simulink model "simulazione"  (R2023a)
settings: Solver=FixedStepAuto  StartTime=0.0  StopTime=10  FixedStep=1e-3  RelTol=1e-3
settings Model: Creator=effi  LastModifiedBy=effi

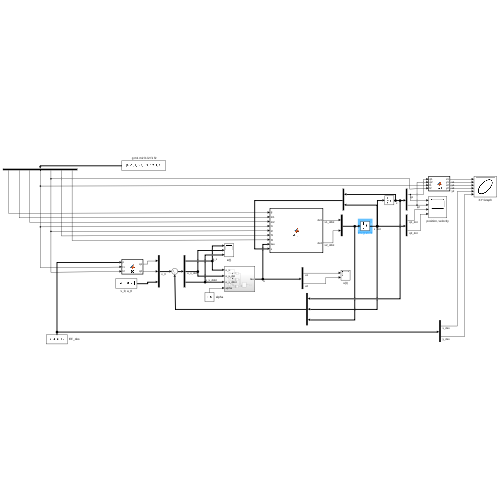
[thumbnail: Simulink's stored preview of the top-level diagram]
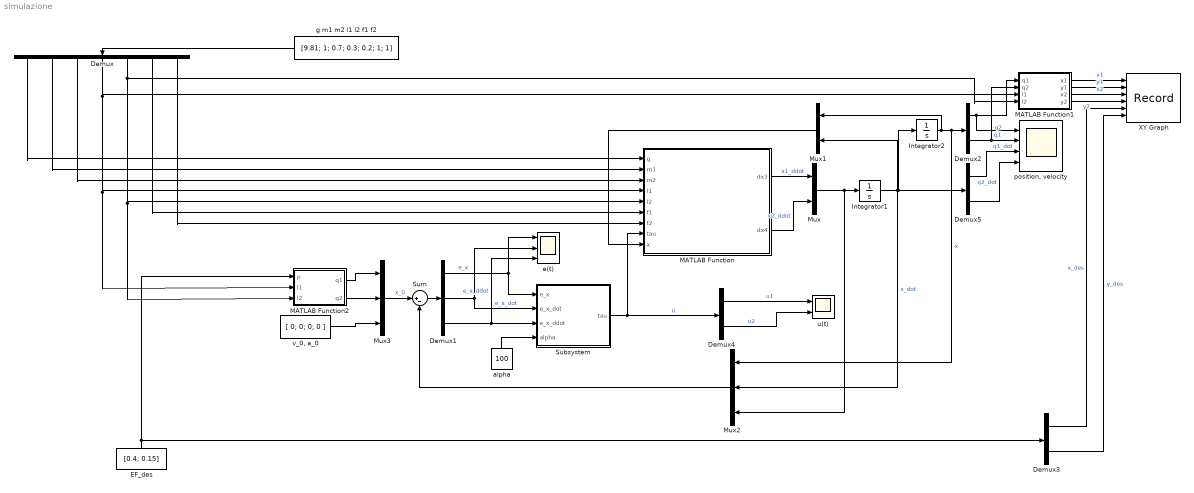
== system simulazione ==
  " g m1 m2 l1 l2 f1 f2" : Constant  Value=[9.81; 1; 0.7; 0.3; 0.2; 1; 1]  SampleTime=-1
  Demux : Demux  Outputs=7
  Demux1 : Demux  Outputs=3
  Demux{2..5} (4 alike) : Demux  Outputs=2
  EF_des : Constant  Value=[0.4; 0.15]  SampleTime=-1
  Integrator1 : Integrator  LimitOutput=on  UpperSaturationLimit=[1;1]*pi/180*20  LowerSaturationLimit=[-1,-1]*pi/180*20
  Integrator2 : Integrator  LimitOutput=on  UpperSaturationLimit=[pi; 5/6*pi]  LowerSaturationLimit=[-pi; -5/6*pi]
  MATLAB Function : MATLAB Function  TreatAsAtomicUnit=on
  MATLAB Function1 : MATLAB Function  TreatAsAtomicUnit=on
  MATLAB Function2 : MATLAB Function  TreatAsAtomicUnit=on
  Mux : Mux  Inputs=2
  Mux1 : Mux  Inputs=2
  Mux2 : Mux  Inputs=3
  Mux3 : Mux  Inputs=3
  Subsystem : Subsystem
  Sum : Sum  Inputs=|+-
  XY Graph : Record  FileSettingsInternal="{\"entries\":[{\"content\":{\"excelSettings\":{\"content\":{},\"type\":\"Streamout.ExcelSettings\"}},\"type\":\"Streamout.FileSettingStorage\",\"uuid\":\"\"}],\"packageUris\":[\"http:\\/\\/schema.mathworks.com\\/mf0\\/streamout_blocks\\/R2020a\"],\"version\":\"1.0\"}"  Layout=[1 1]  SignalsInternal="{\"entries\":[{\"content\":{\"signals\":[{\"content\":{\"blockPath\":[],\"dimensions\":[1],\"domain\":\"\",\"lineColor\":\"#a2142f\",\"plots\":[1],\"port\":1,\"sid\":[\"\"],\"signalID\":10315,\"signalName\":\"x1\"},\"type\":\"RecordBlkView.Signal\",\"uuid\":\"\"},{\"content\":{\"blockPath\":[],\"dimensions\":[1],\"domain\":\"\",\"lineColor\":\"#139fff\",\"plots\":[1],\"port\":2,\"sid\":[\"\"],\"signalID\":10319,\"signalName\":\"y1\"},\"type\":\"RecordBlkView.Signal\",\"uuid\":\"\"},{\"content\":{\"blockPath\":[],\"dimensions\":[1],\"domain\":\"\",\"lineColor\":\"#edb120\",\"plots\":[1],\"port\":3,\"sid\":[\"\"],\"signalID\":10323,\"signalName\":\"x2\"},\"type\":\"RecordBlkView.Signal\",\"uuid\":\"\"},{\"content\":{\"blockPath\":[],\"dimensions\":[1],\"domain\":\"\",\"lineColor\":\"#7e2f8e\",\"plots\":[1],\"port\":4,\"sid\":[\"\"],\"signalID\":10327,\"signalName\":\"y2\"},\"type\":\"RecordBlkView.Signal\",\"uuid\":\"\"},{\"content\":{\"blockPath\":[],\"dimensions\":[1],\"domain\":\"\",\"lineColor\":\"#77ac30\",\"plots\":[1],\"port\":5,\"sid\":[\"\"],\"signalID\":10331,\"signalName\":\"x_des\"},\"type\":\"RecordBlkView.Signal\",\"uuid\":\"\"},{\"content\":{\"blockPath\":[],\"dimensions\":[1],\"domain\":\"\",\"lineColor\":\"#4dbeee\",\"plots\":[1],\"port\":6,\"sid\":[\"\"],\"signalID\":10335,\"signalName\":\"y_des\"},\"type\":\"RecordBlkView.Signal\",\"uuid\":\"\"}]},\"type\":\"RecordBlkView.InputSignals\",\"uuid\":\"\"}],\"packageUris\":[\"http:\\/\\/schema.mathworks.com\\/mf0\\/streamout_blocks\\/R2020a\"],\"version\":\"1.0\"}"  VisualizationBindings="{\"xyplotplugin\":{\"info\":[{\"series\":[{\"bindingParametersList\":[{\"parameter\":\"X-Axis\",\"signalID\":10331,\"signalName\":\"x_des\"},{\"parameter\":\"Y-Axis\",\"signalID\":10335,\"signalName\":\"y_des\"}],\"seriesID\":11819},{\"bindingParametersList\":[{\"parameter\":\"X-Axis\",\"signalID\":10323,\"signalName\":\"x2\"},{\"parameter\":\"Y-Axis\",\"signalID\":10327,\"signalName\":\"y2\"}],\"seriesID\":2499},{\"bindingParametersList\":[{\"parameter\":\"X-Axis\",\"signalID\":10315,\"signalName\":\"x1\"},{\"parameter\":\"Y-Axis\",\"signalID\":10319,\"signalName\":\"y1\"}],\"seriesID\":28857}],\"subplotID\":1}]}}"  CompatibilityTag=XY
  alpha : Constant  Value=100
  e(t) : Scope  NumInputPorts=3
  "position, velocity" : Scope  NumInputPorts=4
  u(t) : Scope  NumInputPorts=2
  "v_0, a_0" : Constant  Value=[ 0; 0; 0; 0 ]  SampleTime=-1
  wires:
  Demux3/2 -> XY Graph/6  "y_des"
  MATLAB Function1/4(y2) -> XY Graph/4  "y2"
  MATLAB Function1/2(y1) -> XY Graph/2  "y1"
  Demux3/1 -> XY Graph/5  "x_des"
  MATLAB Function1/1(x1) -> XY Graph/1  "x1"
  Demux5/2 -> "position, velocity"/4  "q2_dot"
  MATLAB Function1/3(x2) -> XY Graph/3  "x2"
  Demux5/1 -> "position, velocity"/3  "q1_dot"
  " g m1 m2 l1 l2 f1 f2"/1 -> Demux/1
  Subsystem/1(tau) -> Demux4/1, MATLAB Function/8(tau)  "u"
  Demux2/2 -> "position, velocity"/2, MATLAB Function1/2(q2)  "q2"
  EF_des/1 -> MATLAB Function2/1(p), Demux3/1
  Demux/7 -> MATLAB Function/7(f2)
  Demux/1 -> MATLAB Function/1(g)
  Demux4/1 -> u(t)/1  "u1"
  MATLAB Function2/2(q2) -> Mux3/2
  "v_0, a_0"/1 -> Mux3/3
  Demux/4 -> MATLAB Function2/2(l1), MATLAB Function/4(l1), MATLAB Function1/3(l1)
  Integrator2/1 -> Demux2/1, Mux2/1, Mux1/1  "x"
  Demux/5 -> MATLAB Function/5(l2), MATLAB Function2/3(l2), MATLAB Function1/4(l2)
  Mux/1 -> Integrator1/1, Mux2/3
  MATLAB Function2/1(q1) -> Mux3/1
  Demux/3 -> MATLAB Function/3(m2)
  Mux3/1 -> Sum/1  "x_0"
  Integrator1/1 -> Integrator2/1, Demux5/1, Mux2/2, Mux1/2  "x_dot"
  Sum/1 -> Demux1/1
  Demux/2 -> MATLAB Function/2(m1)
  Demux1/3 -> e(t)/3, Subsystem/3(e_x_ddot)  "e_x_ddot"
  alpha/1 -> Subsystem/4(alpha)
  Demux1/1 -> e(t)/1, Subsystem/1(e_x)  "e_x"
  Mux2/1 -> Sum/2
  MATLAB Function/1(dx3) -> Mux/1  "x1_ddot"
  Demux4/2 -> u(t)/2  "u2"
  Demux/6 -> MATLAB Function/6(f1)
  MATLAB Function/2(dx4) -> Mux/2  "x2_ddot"
  Mux1/1 -> MATLAB Function/9(x)
  Demux1/2 -> Subsystem/2(e_x_dot), e(t)/2  "e_x_dot"
  Demux2/1 -> MATLAB Function1/1(q1), "position, velocity"/1  "q1"

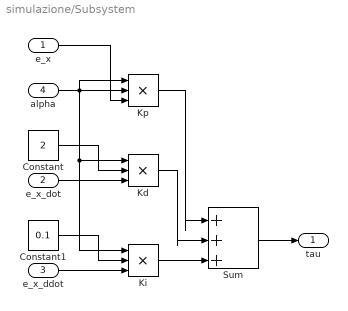
== system simulazione/Subsystem ==
  e_x : Inport
  e_x_dot : Inport  Port=2
  e_x_ddot : Inport  Port=3
  alpha : Inport  Port=4
  Constant : Constant  Value=2
  Constant1 : Constant  Value=0.1
  Kd : Product  Inputs=3
  Ki : Product  Inputs=3
  Kp : Product  Inputs=3
  Sum : Sum  Inputs=|+++
  tau : Outport
  wires:
  Kd/1 -> Sum/2
  Sum/1 -> tau/1
  Constant1/1 -> Ki/2
  Ki/1 -> Sum/3
  e_x_ddot/1 -> Ki/3
  e_x_dot/1 -> Kd/3
  Constant/1 -> Kd/2
  Kp/1 -> Sum/1
  alpha/1 -> Ki/1, Kd/1, Kp/2, Kp/1
  e_x/1 -> Kp/3

== matlab function simulazione/MATLAB Function1 ==
  data: q1 input; x1 output; q2 input; l1 input; l2 input; y1 output; x2 output; y2 output
function [x1,y1,x2,y2] = fwd(q1, q2, l1, l2)

x1 = l1*cos(q1);
y1 = l1*sin(q1);
x2 = x1 + l2*cos(q1+q2);
y2 = y1 + l2*sin(q1+q2);

== matlab function simulazione/MATLAB Function ==
  data: g input; m1 input; m2 input; l1 input; l2 input; f1 input; f2 input; tau input; x input; dx3 output size=1; dx4 output size=1
function [dx3, dx4]  = dxdt(g, m1, m2,l1, l2, f1, f2,tau, x)
    t1 = tau(1);
    t2 = tau(2);
    x1 = x(1);
    x2 = x(2);
    x3 = x(3);
    x4 = x(4);
    % NO FRICTION
    % dx3 = (2*l2*t1 - 2*l2*t2 - 2*l1*t2*cos(x2) - g*l1*l2*m2*cos(x1 + 2*x2) + l1^2*l2*m2*x3^2*sin(2*x2) + 2*l1*l2^2*m2*x3^2*sin(x2) + 2*l1*l2^2*m2*x4^2*sin(x2) + 2*g*l1*l2*m1*cos(x1) + g*l1*l2*m2*cos(x1) + 4*l1*l2^2*m2*x3*x4*sin(x2))/(l1^2*l2*(2*m1 + m2 - m2*cos(2*x2)));
    % dx4 = -(l2^2*m2*t1 - l1^2*m2*t2 - l1^2*m1*t2 - l2^2*m2*t2 + l1*l2^3*m2^2*x3^2*sin(x2) + l1^3*l2*m2^2*x3^2*sin(x2) + l1*l2^3*m2^2*x4^2*sin(x2) + g*l1*l2^2*m2^2*cos(x1) + l1^2*l2^2*m2^2*x3^2*sin(2*x2) + (l1^2*l2^2*m2^2*x4^2*sin(2*x2))/2 + l1*l2*m2*t1*cos(x2) - 2*l1*l2*m2*t2*cos(x2) + l1^3*l2*m1*m2*x3^2*sin(x2) + 2*l1*l2^3*m2^2*x3*x4*sin(x2) + g*l1^2*l2*m2^2*sin(x1)*sin(x2) + g*l1*l2^2*m1*m2*cos(x1) - g*l1*l2^2*m2^2*cos(x1)*cos(x2)^2 + l1^2*l2^2*m2^2*x3*x4*sin(2*x2) + g*l1*l2^2*m2^2*cos(x2)*sin(x1)*sin(x2) + g*l1^2*l2*m1*m2*sin(x1)*sin(x2))/(l1^2*l2^2*m2*(- m2*cos(x2)^2 + m1 + m2));
    % FRICTON
    dx3 = (l2*t1 - l2*t2 - l1*t2*cos(x2) - f1*l2*x3 + f2*l2*x4 + f2*l1*x4*cos(x2) + l1*l2^2*m2*x3^2*sin(x2) + l1*l2^2*m2*x4^2*sin(x2) + g*l1*l2*m1*cos(x1) + g*l1*l2*m2*cos(x1) - g*l1*l2*m2*cos(x1 + x2)*cos(x2) + l1^2*l2*m2*x3^2*cos(x2)*sin(x2) + 2*l1*l2^2*m2*x3*x4*sin(x2))/(l1^2*l2*m1 + l1^2*l2*m2 - l1^2*l2*m2*cos(x2)^2);
    dx4 = -(l2^2*m2*t1 - l1^2*m2*t2 - l1^2*m1*t2 - l2^2*m2*t2 - f1*l2^2*m2*x3 + f2*l1^2*m1*x4 + f2*l1^2*m2*x4 + f2*l2^2*m2*x4 + l1*l2^3*m2^2*x3^2*sin(x2) + l1^3*l2*m2^2*x3^2*sin(x2) + l1*l2^3*m2^2*x4^2*sin(x2) - g*l1^2*l2*m2^2*cos(x1 + x2) + g*l1*l2^2*m2^2*cos(x1) + l1*l2*m2*t1*cos(x2) - 2*l1*l2*m2*t2*cos(x2) + l1^3*l2*m1*m2*x3^2*sin(x2) + 2*l1*l2^3*m2^2*x3*x4*sin(x2) - g*l1*l2^2*m2^2*cos(x1 + x2)*cos(x2) - f1*l1*l2*m2*x3*cos(x2) + 2*f2*l1*l2*m2*x4*cos(x2) + 2*l1^2*l2^2*m2^2*x3^2*cos(x2)*sin(x2) + l1^2*l2^2*m2^2*x4^2*cos(x2)*sin(x2) + g*l1^2*l2*m2^2*cos(x1)*cos(x2) - g*l1^2*l2*m1*m2*cos(x1 + x2) + g*l1*l2^2*m1*m2*cos(x1) + 2*l1^2*l2^2*m2^2*x3*x4*cos(x2)*sin(x2) + g*l1^2*l2*m1*m2*cos(x1)*cos(x2))/(- l1^2*l2^2*m2^2*cos(x2)^2 + l1^2*l2^2*m2^2 + m1*l1^2*l2^2*m2);
end

== matlab function simulazione/MATLAB Function2 ==
  data: p input; q1 output; l1 input; l2 input; q2 output
function [q1, q2] = IK(p, l1, l2)
XE = p(1);
YE = p(2);
c2 = (XE^2+YE^2-l1^2-l2^2)/(2*l1*l2);
s2 = sqrt(1-c2^2);
q2 = atan2(s2,c2);
R2 = [c2, -s2; s2, c2];
RHS = R2*[l2;0]+[l1;0];
a = RHS(1);
b = RHS(2);
LHS = 1/(a^2+b^2)*[a b; -b a]*[XE; YE];
c1 = LHS(1);
s1 = LHS(2);
q1 = atan2(s1,c1);
